simulink model "ModeAdjust"  (R2018b)
settings: Solver=FixedStepDiscrete  StartTime=0.0  StopTime=inf  FixedStep=0.01  RelTol=1e-3
undefined symbols (not defined in the file or in its folder): IfKeSMSbSeatMovBkRclnEnable_Val, IfKeSMSbSeatMovFrwdBkwdEnable_Val, IfKeSMSbSeatMovFtrstEnable_Val, IfKeSMSbSeatMovHdrstFrwdBkwdEnable_Val, IfKeSMSbSeatMovHdUpwdDnwdEnable_Val, IfKeSMSbSeatMovLgrstEnable_Val, IfKeSMSbSeatMovLtwdRtwdEnable_Val, IfVeSMSeStNumConfig, KeSMSbArmscreenMovEnable_Val, KeSMSbSeatMovLgrstExpdEnable_Val, KeSMSuFirstRwStBackPosDelta_Val, KeSMSuFirstRwStBackPosTolr_Val, KeSMSuFirstRwStCushFrntPosDelta_Val, KeSMSuFirstRwStCushFrntPosTolr_Val, KeSMSuFirstRwStCushRePosDelta_Val, KeSMSuFirstRwStCushRePosTolr_Val, KeSMSuFirstRwStFootrestPosDelta_Val, KeSMSuFirstRwStFootrestPosTolr_Val, KeSMSuFirstRwStFwdBkwdPosDelta_Val, KeSMSuFirstRwStFwdBkwdPosTolr_Val, KeSMSuMdMotFinshdTm_Val, KeSMSuMdRetryTm1_Val, KeSMSuModeReqDurgTm_Val, KeSMSuSecRwStArmTochPosDelta_Val, KeSMSuSecRwStArmTochPosTolr_Val, KeSMSuSecRwStBackPosDelta_Val, KeSMSuSecRwStBackPosTolr_Val, KeSMSuSecRwStFtrstUpwdDnwdPosDelta_Val, KeSMSuSecRwStFtrstUpwdDnwdPosTolr_Val, KeSMSuSecRwStFwdBkwdPosDelta_Val, KeSMSuSecRwStFwdBkwdPosTolr_Val, KeSMSuSecRwStHeadrestFwdBkwdPosDelta_Val, KeSMSuSecRwStHeadrestFwdBkwdPosTolr_Val, KeSMSuSecRwStHeadrestUpwdDwnwdPosDelta_Val, KeSMSuSecRwStHeadrestUpwdDwnwdPosTolr_Val, KeSMSuSecRwStLegrestInOutPosDelta_Val, KeSMSuSecRwStLegrestInOutPosTolr_Val, KeSMSuSecRwStLegrestUpwdDwnwdPosDelta_Val, KeSMSuSecRwStLegrestUpwdDwnwdPosTolr_Val, KeSMSuSecRwStLwdRwdPosDelta_Val, KeSMSuSecRwStLwdRwdPosTolr_Val, KeSMSuSecRwStVIPFtrstRefAngle_Val, KeSMSuThirdRwStFwdBkwdPosDelta_Val, KeSMSuThirdRwStFwdBkwdPosTolr_Val, KeSMSuThrdRwCushFoldPosDelta_Val, KeSMSuThrdRwCushFoldPosTolr_Val, KeSMSuThrdRwStBackPosDelta_Val, KeSMSuThrdRwStBackPosTolr_Val, KeSMSw4SLegrstCloseMdSecRwLtStFtrstUpwdDnwdPos_Val, KeSMSw4SLegrstCloseMdSecRwLtStFtrstUpwdDnwdPosMax_Val, KeSMSw4SLegrstCloseMdSecRwLtStFtrstUpwdDnwdPosMin_Val, KeSMSw4SLegrstCloseMdSecRwLtStLgrstOtwdInwdPos_Val, KeSMSw4SLegrstCloseMdSecRwLtStLgrstOtwdInwdPosMax_Val, KeSMSw4SLegrstCloseMdSecRwLtStLgrstOtwdInwdPosMin_Val, KeSMSw4SLegrstCloseMdSecRwLtStLgrstUpwdDnwdPos_Val, KeSMSw4SLegrstCloseMdSecRwLtStLgrstUpwdDnwdPosMax_Val, KeSMSw4SLegrstCloseMdSecRwLtStLgrstUpwdDnwdPosMin_Val, KeSMSw4SLegrstCloseMdSecRwRtStFtrstUpwdDnwdPos_Val, KeSMSw4SLegrstCloseMdSecRwRtStFtrstUpwdDnwdPosMax_Val, KeSMSw4SLegrstCloseMdSecRwRtStFtrstUpwdDnwdPosMin_Val ... (+1138)
libraries: Lib x401
(part 33 of 35)

== system ModeAdjust/ModeAdjustRunnable_sys/ModeAdjust/ArrivedAtTargetPosChk/Vip4s/R2Rt ==
  SecRwLtStsPoss : Inport
  ModeStCalib_2L : Inport  Port=2
  StConfig : Inport  Port=3
  SecRwLtStsPoss4s : Inport  Port=4
  StConfig4s : Inport  Port=5
  SecRwRtStPossV : Inport  Port=6
  PosV4s : Inport  Port=7
  Rt4sHightIndex : Inport  Port=8
  PosDeltaCalib : Inport  Port=9
  Bus Creator{1..7} (7 alike) : BusCreator  Inputs=9
  Bus Selector : BusSelector  OutputSignals=IfVeSMSuSecRwRtStBkReclnUpwdDnwdPos_Val_read,IfVeSMSuSecRwRtStFrwdBkwdPos_Val_read,IfVeSMSuSecRwRtStHPassStUpwdDnwdPos_Val_read,IfVeSMSuSecRwRtStLgrstUpwdDnwdPos_Val_read,IfVeSMSuSecRwRtStLtwdRtwdPos_Val_read,SecRwRtStArmScrnPos_Val_read
  Bus Selector1 : BusSelector  OutputSignals=IfVeSMSuSecRwRtStLgrstOtwdInwdPos_Val_read,IfVeSMSuRrRtStFtUpwdDnwdPos_Val_read,IfVeSMSuSecRwRtStHdrstFrwdBkwdPos_Val_read
  Bus Selector2 : BusSelector  OutputSignals=BkReclnUpwdDnwdPos,BkReclnUpwdDnwdPosMax,BkReclnUpwdDnwdPosMin,LgrstUpwdPos,LgrstUpwdPosMax,LgrstUpwdPosMin,FtrstUpwdDnwdPos,FtrstUpwdDnwdPosMax,FtrstUpwdDnwdPosMin
  Bus Selector3 : BusSelector  OutputSignals=VipRSecRwRtSt
  Bus Selector4 : BusSelector  OutputSignals=BkReclnUpwdDnwdMovConfig,ArmTouchMovConfig,FrwdBkwdMovConfig,LgrstUpwdMovConfig,LtwdRtwdMovConfig
  Bus Selector5 : BusSelector  OutputSignals=LgrstExpdMovConfig,FtrstMovConfig,HdrstUpwdDnwdMovConfig,HdrstFrwdBkwdMovConfig
  Bus Selector6 : BusSelector  OutputSignals=IfVeSMSuSecRwRtStBkReclnUpwdDnwdPosV_Val_read,IfVeSMSuSecRwRtStFrwdBkwdPosV_Val_read,IfVeSMSuSecRwRtStHPassStUpwdDnwdPosV_Val_read,IfVeSMSuSecRwRtStLgrstUpwdDnwdPosV_Val_read,IfVeSMSuSecRwRtStLtwdRtwdPosV_Val_read,SecRwRtStArmScrnPosV_Val_read
  Bus Selector7 : BusSelector  OutputSignals=IfVeSMSuSecRwRtStLgrstOtwdInwdPosV_Val_read,IfVeSMSuRrRtStFtUpwdDnwdPosV_Val_read,IfVeSMSuSecRwRtStHdrstFrwdBkwdPosV_Val_read
  Bus Selector8 : BusSelector  OutputSignals=HdrstUpwdDnwdPosMax,HdrstUpwdDnwdPosMin,LgrstOtwdInwdPosMax,LgrstOtwdInwdPosMin,HdrstFrwdBkwdnwdPosMax,HdrstFrwdBkwdnwdPosMin
  Bus Selector9 : BusSelector  OutputSignals=KeSMSuSecRwStHeadrestFwdBkwdPosDelta_Val,KeSMSuSecRwStHeadrestUpwdDwnwdPosDelta_Val,KeSMSuSecRwStLegrestInOutPosDelta_Val,KeSMSuSecRwStFtrstUpwdDnwdPosDelta_Val,KeSMSuSecRwStBackPosDelta_Val,KeSMSuSecRwStLegrestUpwdDwnwdPosDelta_Val
  CheckAtPos{,1..5} (6 alike) : Lib/CheckAtPos  SystemSampleTime=-1
  Constant{1..12} (12 alike) : Constant  Value=0  OutDataTypeStr=boolean
  IsArrivedTarZone{,1..5} (6 alike) : Lib/CommonUsed/IniPosjudg/Subsystem2  SystemSampleTime=-1
  Logical Operator9 : Logic  Inputs=6  AllPortsSameDT=off  OutDataTypeStr=boolean
  Multiport Switch : MultiPortSwitch  DataPortOrder=Zero-based contiguous  Inputs=7  DiagnosticForDefault=None  zeroidx=on
  PA_KeSMSw4sVIPMDSecRwRtStHdrstFrwdBkwdPosMax_160_Val : Constant  Value=KeSMSw4sVIPMDSecRwRtStHdrstFrwdBkwdPosMax_160_Val
  PA_KeSMSw4sVIPMDSecRwRtStHdrstFrwdBkwdPosMax_165_Val : Constant  Value=KeSMSw4sVIPMDSecRwRtStHdrstFrwdBkwdPosMax_165_Val
  PA_KeSMSw4sVIPMDSecRwRtStHdrstFrwdBkwdPosMax_170_Val : Constant  Value=KeSMSw4sVIPMDSecRwRtStHdrstFrwdBkwdPosMax_170_Val
  PA_KeSMSw4sVIPMDSecRwRtStHdrstFrwdBkwdPosMax_175_Val : Constant  Value=KeSMSw4sVIPMDSecRwRtStHdrstFrwdBkwdPosMax_175_Val
  PA_KeSMSw4sVIPMDSecRwRtStHdrstFrwdBkwdPosMax_180_Val : Constant  Value=KeSMSw4sVIPMDSecRwRtStHdrstFrwdBkwdPosMax_180_Val
  PA_KeSMSw4sVIPMDSecRwRtStHdrstFrwdBkwdPosMax_Below160_Val : Constant  Value=KeSMSw4sVIPMDSecRwRtStHdrstFrwdBkwdPosMax_Below160_Val
  PA_KeSMSw4sVIPMDSecRwRtStHdrstFrwdBkwdPosMax_Over180_Val : Constant  Value=KeSMSw4sVIPMDSecRwRtStHdrstFrwdBkwdPosMax_Over180_Val
  PA_KeSMSw4sVIPMDSecRwRtStHdrstFrwdBkwdPosMin_160_Val : Constant  Value=KeSMSw4sVIPMDSecRwRtStHdrstFrwdBkwdPosMin_160_Val
  PA_KeSMSw4sVIPMDSecRwRtStHdrstFrwdBkwdPosMin_165_Val : Constant  Value=KeSMSw4sVIPMDSecRwRtStHdrstFrwdBkwdPosMin_165_Val
  PA_KeSMSw4sVIPMDSecRwRtStHdrstFrwdBkwdPosMin_170_Val : Constant  Value=KeSMSw4sVIPMDSecRwRtStHdrstFrwdBkwdPosMin_170_Val
  PA_KeSMSw4sVIPMDSecRwRtStHdrstFrwdBkwdPosMin_175_Val : Constant  Value=KeSMSw4sVIPMDSecRwRtStHdrstFrwdBkwdPosMin_175_Val
  PA_KeSMSw4sVIPMDSecRwRtStHdrstFrwdBkwdPosMin_180_Val : Constant  Value=KeSMSw4sVIPMDSecRwRtStHdrstFrwdBkwdPosMin_180_Val
  PA_KeSMSw4sVIPMDSecRwRtStHdrstFrwdBkwdPosMin_Below160_Val : Constant  Value=KeSMSw4sVIPMDSecRwRtStHdrstFrwdBkwdPosMin_Below160_Val
  PA_KeSMSw4sVIPMDSecRwRtStHdrstFrwdBkwdPosMin_Over180_Val : Constant  Value=KeSMSw4sVIPMDSecRwRtStHdrstFrwdBkwdPosMin_Over180_Val
  PA_KeSMSw4sVIPMDSecRwRtStHdrstFrwdBkwdPos_160_Val : Constant  Value=KeSMSw4sVIPMDSecRwRtStHdrstFrwdBkwdPos_160_Val
  PA_KeSMSw4sVIPMDSecRwRtStHdrstFrwdBkwdPos_165_Val : Constant  Value=KeSMSw4sVIPMDSecRwRtStHdrstFrwdBkwdPos_165_Val
  PA_KeSMSw4sVIPMDSecRwRtStHdrstFrwdBkwdPos_170_Val : Constant  Value=KeSMSw4sVIPMDSecRwRtStHdrstFrwdBkwdPos_170_Val
  PA_KeSMSw4sVIPMDSecRwRtStHdrstFrwdBkwdPos_175_Val : Constant  Value=KeSMSw4sVIPMDSecRwRtStHdrstFrwdBkwdPos_175_Val
  PA_KeSMSw4sVIPMDSecRwRtStHdrstFrwdBkwdPos_180_Val : Constant  Value=KeSMSw4sVIPMDSecRwRtStHdrstFrwdBkwdPos_180_Val
  PA_KeSMSw4sVIPMDSecRwRtStHdrstFrwdBkwdPos_Below160_Val : Constant  Value=KeSMSw4sVIPMDSecRwRtStHdrstFrwdBkwdPos_Below160_Val
  PA_KeSMSw4sVIPMDSecRwRtStHdrstFrwdBkwdPos_Over180_Val : Constant  Value=KeSMSw4sVIPMDSecRwRtStHdrstFrwdBkwdPos_Over180_Val
  PA_KeSMSw4sVIPMDSecRwRtStHdrstUpwdPosMax_160_Val : Constant  Value=KeSMSw4sVIPMDSecRwRtStHdrstUpwdPosMax_160_Val
  PA_KeSMSw4sVIPMDSecRwRtStHdrstUpwdPosMax_165_Val : Constant  Value=KeSMSw4sVIPMDSecRwRtStHdrstUpwdPosMax_165_Val
  PA_KeSMSw4sVIPMDSecRwRtStHdrstUpwdPosMax_170_Val : Constant  Value=KeSMSw4sVIPMDSecRwRtStHdrstUpwdPosMax_170_Val
  PA_KeSMSw4sVIPMDSecRwRtStHdrstUpwdPosMax_175_Val : Constant  Value=KeSMSw4sVIPMDSecRwRtStHdrstUpwdPosMax_175_Val
  PA_KeSMSw4sVIPMDSecRwRtStHdrstUpwdPosMax_180_Val : Constant  Value=KeSMSw4sVIPMDSecRwRtStHdrstUpwdPosMax_180_Val
  PA_KeSMSw4sVIPMDSecRwRtStHdrstUpwdPosMax_Below160_Val : Constant  Value=KeSMSw4sVIPMDSecRwRtStHdrstUpwdPosMax_Below160_Val
  PA_KeSMSw4sVIPMDSecRwRtStHdrstUpwdPosMax_Over180_Val : Constant  Value=KeSMSw4sVIPMDSecRwRtStHdrstUpwdPosMax_Over180_Val
  PA_KeSMSw4sVIPMDSecRwRtStHdrstUpwdPosMin_160_Val : Constant  Value=KeSMSw4sVIPMDSecRwRtStHdrstUpwdPosMin_160_Val
  PA_KeSMSw4sVIPMDSecRwRtStHdrstUpwdPosMin_165_Val : Constant  Value=KeSMSw4sVIPMDSecRwRtStHdrstUpwdPosMin_165_Val
  PA_KeSMSw4sVIPMDSecRwRtStHdrstUpwdPosMin_170_Val : Constant  Value=KeSMSw4sVIPMDSecRwRtStHdrstUpwdPosMin_170_Val
  PA_KeSMSw4sVIPMDSecRwRtStHdrstUpwdPosMin_175_Val : Constant  Value=KeSMSw4sVIPMDSecRwRtStHdrstUpwdPosMin_175_Val
  PA_KeSMSw4sVIPMDSecRwRtStHdrstUpwdPosMin_180_Val : Constant  Value=KeSMSw4sVIPMDSecRwRtStHdrstUpwdPosMin_180_Val
  PA_KeSMSw4sVIPMDSecRwRtStHdrstUpwdPosMin_Below160_Val : Constant  Value=KeSMSw4sVIPMDSecRwRtStHdrstUpwdPosMin_Below160_Val
  PA_KeSMSw4sVIPMDSecRwRtStHdrstUpwdPosMin_Over180_Val : Constant  Value=KeSMSw4sVIPMDSecRwRtStHdrstUpwdPosMin_Over180_Val
  PA_KeSMSw4sVIPMDSecRwRtStHdrstUpwdPos_160_Val : Constant  Value=KeSMSw4sVIPMDSecRwRtStHdrstUpwdPos_160_Val
  PA_KeSMSw4sVIPMDSecRwRtStHdrstUpwdPos_165_Val : Constant  Value=KeSMSw4sVIPMDSecRwRtStHdrstUpwdPos_165_Val
  PA_KeSMSw4sVIPMDSecRwRtStHdrstUpwdPos_170_Val : Constant  Value=KeSMSw4sVIPMDSecRwRtStHdrstUpwdPos_170_Val
  PA_KeSMSw4sVIPMDSecRwRtStHdrstUpwdPos_175_Val : Constant  Value=KeSMSw4sVIPMDSecRwRtStHdrstUpwdPos_175_Val
  PA_KeSMSw4sVIPMDSecRwRtStHdrstUpwdPos_180_Val : Constant  Value=KeSMSw4sVIPMDSecRwRtStHdrstUpwdPos_180_Val
  PA_KeSMSw4sVIPMDSecRwRtStHdrstUpwdPos_Below160_Val : Constant  Value=KeSMSw4sVIPMDSecRwRtStHdrstUpwdPos_Below160_Val
  PA_KeSMSw4sVIPMDSecRwRtStHdrstUpwdPos_Over180_Val : Constant  Value=KeSMSw4sVIPMDSecRwRtStHdrstUpwdPos_Over180_Val
  PA_KeSMSw4sVIPMDSecRwRtStLgrstOtwdInwdPosMax_160_Val : Constant  Value=KeSMSw4sVIPMDSecRwRtStLgrstOtwdInwdPosMax_160_Val
  PA_KeSMSw4sVIPMDSecRwRtStLgrstOtwdInwdPosMax_165_Val : Constant  Value=KeSMSw4sVIPMDSecRwRtStLgrstOtwdInwdPosMax_165_Val
  PA_KeSMSw4sVIPMDSecRwRtStLgrstOtwdInwdPosMax_170_Val : Constant  Value=KeSMSw4sVIPMDSecRwRtStLgrstOtwdInwdPosMax_170_Val
  PA_KeSMSw4sVIPMDSecRwRtStLgrstOtwdInwdPosMax_175_Val : Constant  Value=KeSMSw4sVIPMDSecRwRtStLgrstOtwdInwdPosMax_175_Val
  PA_KeSMSw4sVIPMDSecRwRtStLgrstOtwdInwdPosMax_180_Val : Constant  Value=KeSMSw4sVIPMDSecRwRtStLgrstOtwdInwdPosMax_180_Val
  PA_KeSMSw4sVIPMDSecRwRtStLgrstOtwdInwdPosMax_Below160_Val : Constant  Value=KeSMSw4sVIPMDSecRwRtStLgrstOtwdInwdPosMax_Below160_Val
  PA_KeSMSw4sVIPMDSecRwRtStLgrstOtwdInwdPosMax_Over180_Val : Constant  Value=KeSMSw4sVIPMDSecRwRtStLgrstOtwdInwdPosMax_Over180_Val
  PA_KeSMSw4sVIPMDSecRwRtStLgrstOtwdInwdPosMin_160_Val : Constant  Value=KeSMSw4sVIPMDSecRwRtStLgrstOtwdInwdPosMin_160_Val
  PA_KeSMSw4sVIPMDSecRwRtStLgrstOtwdInwdPosMin_165_Val : Constant  Value=KeSMSw4sVIPMDSecRwRtStLgrstOtwdInwdPosMin_165_Val
  PA_KeSMSw4sVIPMDSecRwRtStLgrstOtwdInwdPosMin_170_Val : Constant  Value=KeSMSw4sVIPMDSecRwRtStLgrstOtwdInwdPosMin_170_Val
  PA_KeSMSw4sVIPMDSecRwRtStLgrstOtwdInwdPosMin_175_Val : Constant  Value=KeSMSw4sVIPMDSecRwRtStLgrstOtwdInwdPosMin_175_Val
  PA_KeSMSw4sVIPMDSecRwRtStLgrstOtwdInwdPosMin_180_Val : Constant  Value=KeSMSw4sVIPMDSecRwRtStLgrstOtwdInwdPosMin_180_Val
  PA_KeSMSw4sVIPMDSecRwRtStLgrstOtwdInwdPosMin_Below160_Val : Constant  Value=KeSMSw4sVIPMDSecRwRtStLgrstOtwdInwdPosMin_Below160_Val
  PA_KeSMSw4sVIPMDSecRwRtStLgrstOtwdInwdPosMin_Over180_Val : Constant  Value=KeSMSw4sVIPMDSecRwRtStLgrstOtwdInwdPosMin_Over180_Val
  PA_KeSMSw4sVIPMDSecRwRtStLgrstOtwdInwdPos_160_Val : Constant  Value=KeSMSw4sVIPMDSecRwRtStLgrstOtwdInwdPos_160_Val
  PA_KeSMSw4sVIPMDSecRwRtStLgrstOtwdInwdPos_165_Val : Constant  Value=KeSMSw4sVIPMDSecRwRtStLgrstOtwdInwdPos_165_Val
  PA_KeSMSw4sVIPMDSecRwRtStLgrstOtwdInwdPos_170_Val : Constant  Value=KeSMSw4sVIPMDSecRwRtStLgrstOtwdInwdPos_170_Val
  PA_KeSMSw4sVIPMDSecRwRtStLgrstOtwdInwdPos_175_Val : Constant  Value=KeSMSw4sVIPMDSecRwRtStLgrstOtwdInwdPos_175_Val
  PA_KeSMSw4sVIPMDSecRwRtStLgrstOtwdInwdPos_180_Val : Constant  Value=KeSMSw4sVIPMDSecRwRtStLgrstOtwdInwdPos_180_Val
  PA_KeSMSw4sVIPMDSecRwRtStLgrstOtwdInwdPos_Below160_Val : Constant  Value=KeSMSw4sVIPMDSecRwRtStLgrstOtwdInwdPos_Below160_Val
  PA_KeSMSw4sVIPMDSecRwRtStLgrstOtwdInwdPos_Over180_Val : Constant  Value=KeSMSw4sVIPMDSecRwRtStLgrstOtwdInwdPos_Over180_Val
  R2Lt_ArrivedTarPos : Outport
  Calib_VIP4sRAdpt : Outport  Port=2
  wires:
  IsArrivedTarZone/1 -> [Step1_1_ArrivedTarPos]
  [SecRwLtStBkReclnUpwdDnwdPos] -> IsArrivedTarZone/1
  [K_BkReclnUpwdDnwdPosMin] -> IsArrivedTarZone/2
  Bus Selector/5 -> [SecRwLtStLtwdRtwdPos]  "<IfVeSMSuSecRwRtStLtwdRtwdPos_Val_read>"
  SecRwLtStsPoss/1 -> Bus Selector/1
  Bus Selector/3 -> [SecRwLtStHPassStUpwdDnwdPos]  "<IfVeSMSuSecRwRtStHPassStUpwdDnwdPos_Val_read>"
  Bus Selector/4 -> [SecRwLtStLgrstUpwdDnwdPos]  "<IfVeSMSuSecRwRtStLgrstUpwdDnwdPos_Val_read>"
  Bus Selector/2 -> [SecRwLtStFrwdBkwdPos]  "<IfVeSMSuSecRwRtStFrwdBkwdPos_Val_read>"
  Bus Selector/1 -> [SecRwLtStBkReclnUpwdDnwdPos]  "<IfVeSMSuSecRwRtStBkReclnUpwdDnwdPos_Val_read>"
  [K_LgrstUpwdPosMin] -> IsArrivedTarZone1/2
  [SecRwLtStLgrstUpwdDnwdPos] -> IsArrivedTarZone1/1
  IsArrivedTarZone1/1 -> [Step1_2_ArrivedTarPos]
  Logical Operator9/1 -> R2Lt_ArrivedTarPos/1
  IsArrivedTarZone2/1 -> [Step1_3_ArrivedTarPos]
  Bus Selector/6 -> [SecRwLtStArmScrnPos]  "<SecRwRtStArmScrnPos_Val_read>"
  [KeSMSuSecRwStBackPosDelta_Val] -> IsArrivedTarZone/3
  [K_BkReclnUpwdDnwdPosMax] -> IsArrivedTarZone/4
  [K_LgrstUpwdPosMax] -> IsArrivedTarZone1/4
  [KeSMSuSecRwStLegrestUpwdDwnwdPosDelta_Val] -> IsArrivedTarZone1/3
  Bus Selector2/6 -> [K_LgrstUpwdPosMin]  "<LgrstUpwdPosMin>"
  Bus Selector2/4 -> [K_LgrstUpwdPos]  "<LgrstUpwdPos>"
  Bus Selector2/5 -> [K_LgrstUpwdPosMax]  "<LgrstUpwdPosMax>"
  Bus Selector2/1 -> [K_BkReclnUpwdDnwdPos]  "<BkReclnUpwdDnwdPos>"
  Bus Selector2/2 -> [K_BkReclnUpwdDnwdPosMax]  "<BkReclnUpwdDnwdPosMax>"
  Bus Selector3/1 -> Bus Selector2/1  "<VipRSecRwRtSt>"
  Bus Selector2/3 -> [K_BkReclnUpwdDnwdPosMin]  "<BkReclnUpwdDnwdPosMin>"
  ModeStCalib_2L/1 -> Bus Selector3/1
  StConfig/1 -> Bus Selector4/1
  Bus Selector4/3 -> [FrwdBkwdMovConfig]  "<FrwdBkwdMovConfig>"
  Bus Selector4/5 -> [LtwdRtwdMovConfig]  "<LtwdRtwdMovConfig>"
  Bus Selector4/4 -> [LgrstUpwdMovConfig]  "<LgrstUpwdMovConfig>"
  Bus Selector4/2 -> [ArmTouchMovConfig]  "<ArmTouchMovConfig>"
  Bus Selector4/1 -> [BkReclnUpwdDnwdMovConfig]  "<BkReclnUpwdDnwdMovConfig>"
  [K_HdrstUpwdPosMax] -> IsArrivedTarZone2/4
  [K_HdrstUpwdPosMin] -> IsArrivedTarZone2/2
  [SecRwLtStHPassStUpwdDnwdPos] -> IsArrivedTarZone2/1
  [KeSMSuSecRwStHeadrestUpwdDwnwdPosDelta_Val] -> IsArrivedTarZone2/3
  [KeSMSuSecRwStFtrstUpwdDnwdPosDelta_Val] -> IsArrivedTarZone3/3
  SecRwLtStsPoss4s/1 -> Bus Selector1/1
  Bus Selector1/1 -> [SecRwLtStLgrstOtwdInwdPos]  "<IfVeSMSuSecRwRtStLgrstOtwdInwdPos_Val_read>"
  Bus Selector1/2 -> [IfVeSMSuRrLtStFtUpwdDnwdPos]  "<IfVeSMSuRrRtStFtUpwdDnwdPos_Val_read>"
  [IfVeSMSuRrLtStFtUpwdDnwdPos] -> IsArrivedTarZone3/1
  Bus Selector2/7 -> [K_FtrstUpwdDnwdPos]  "<FtrstUpwdDnwdPos>"
  Bus Selector2/8 -> [K_FtrstUpwdDnwdPos_Max]  "<FtrstUpwdDnwdPosMax>"
  Bus Selector2/9 -> [K_FtrstUpwdDnwdPos_Min]  "<FtrstUpwdDnwdPosMin>"
  [K_FtrstUpwdDnwdPos_Min] -> IsArrivedTarZone3/2
  [K_FtrstUpwdDnwdPos_Max] -> IsArrivedTarZone3/4
  IsArrivedTarZone3/1 -> [Step1_4_ArrivedTarPos]
  [K_LgrstOtwdInwdPos_Min] -> IsArrivedTarZone4/2
  [K_LgrstOtwdInwdPos_Max] -> IsArrivedTarZone4/4
  [SecRwLtStLgrstOtwdInwdPos] -> IsArrivedTarZone4/1
  [KeSMSuSecRwStLegrestInOutPosDelta_Val] -> IsArrivedTarZone4/3
  IsArrivedTarZone4/1 -> [Step1_5_ArrivedTarPos]
  StConfig4s/1 -> Bus Selector5/1
  Bus Selector5/3 -> [HdrstMovConfig]  "<HdrstUpwdDnwdMovConfig>"
  Bus Selector5/1 -> [LgrstExpdMovConfig]  "<LgrstExpdMovConfig>"
  Bus Selector5/2 -> [FtrstMovConfig]  "<FtrstMovConfig>"
  PosV4s/1 -> Bus Selector7/1
  Bus Selector7/2 -> [RrLtStFtUpwdDnwdPosV]  "<IfVeSMSuRrRtStFtUpwdDnwdPosV_Val_read>"
  Bus Selector7/1 -> [SecRwLtStLgrstOtwdInwdPosV]  "<IfVeSMSuSecRwRtStLgrstOtwdInwdPosV_Val_read>"
  Bus Selector6/5 -> [SecRwRtStLtwdRtwdPosV]  "<IfVeSMSuSecRwRtStLtwdRtwdPosV_Val_read>"
  SecRwRtStPossV/1 -> Bus Selector6/1
  Bus Selector6/6 -> [SecRwRtStArmScrnPosV]  "<SecRwRtStArmScrnPosV_Val_read>"
  Bus Selector6/3 -> [SecRwRtStHPassStUpwdDnwdPosV]  "<IfVeSMSuSecRwRtStHPassStUpwdDnwdPosV_Val_read>"
  Bus Selector6/4 -> [SecRwRtStLgrstUpwdDnwdPosV]  "<IfVeSMSuSecRwRtStLgrstUpwdDnwdPosV_Val_read>"
  Bus Selector6/2 -> [SecRwRtStFrwdBkwdPosV]  "<IfVeSMSuSecRwRtStFrwdBkwdPosV_Val_read>"
  Bus Selector6/1 -> [SecRwRtStBkReclnUpwdDnwdPosV]  "<IfVeSMSuSecRwRtStBkReclnUpwdDnwdPosV_Val_read>"
  CheckAtPos2/1 -> Logical Operator9/3  "Vip4sR_Step1_3_ArrivedTarPos"
  CheckAtPos1/1 -> Logical Operator9/2  "Vip4sR_Step1_2_ArrivedTarPos"
  CheckAtPos3/1 -> Logical Operator9/4  "Vip4sR_Step1_4_ArrivedTarPos"
  CheckAtPos/1 -> Logical Operator9/1  "Vip4sR_Step1_1_ArrivedTarPos"
  CheckAtPos4/1 -> Logical Operator9/5  "Vip4sR_Step1_5_ArrivedTarPos"
  [BkReclnUpwdDnwdMovConfig] -> CheckAtPos/1
  [Step1_1_ArrivedTarPos] -> CheckAtPos/3
  [LgrstUpwdMovConfig] -> CheckAtPos1/1
  [Step1_2_ArrivedTarPos] -> CheckAtPos1/3
  [HdrstMovConfig] -> CheckAtPos2/1
  [Step1_3_ArrivedTarPos] -> CheckAtPos2/3
  [FtrstMovConfig] -> CheckAtPos3/1
  [Step1_4_ArrivedTarPos] -> CheckAtPos3/3
  [LgrstExpdMovConfig] -> CheckAtPos4/1
  [Step1_5_ArrivedTarPos] -> CheckAtPos4/3
  Constant8/1 -> CheckAtPos4/4
  Constant7/1 -> CheckAtPos4/5
  Constant2/1 -> CheckAtPos3/4
  Constant1/1 -> CheckAtPos3/5
  Constant4/1 -> CheckAtPos2/4
  Constant3/1 -> CheckAtPos2/5
  Constant6/1 -> CheckAtPos1/4
  Constant5/1 -> CheckAtPos1/5
  Constant12/1 -> CheckAtPos/4
  Constant11/1 -> CheckAtPos/5
  [SecRwRtStBkReclnUpwdDnwdPosV] -> CheckAtPos/2
  [SecRwRtStLgrstUpwdDnwdPosV] -> CheckAtPos1/2
  [SecRwRtStHPassStUpwdDnwdPosV] -> CheckAtPos2/2
  [RrLtStFtUpwdDnwdPosV] -> CheckAtPos3/2
  [SecRwLtStLgrstOtwdInwdPosV] -> CheckAtPos4/2
  Bus Selector5/4 -> [HdrstFrwdBkwdMovConfig]  "<HdrstFrwdBkwdMovConfig>"
  [SecRwRtStHdrstFrwdBkwdPos] -> IsArrivedTarZone5/1
  [HdrstFrwdBkwdMovConfig] -> CheckAtPos5/1
  [Step1_6_ArrivedTarPos] -> CheckAtPos5/3
  IsArrivedTarZone5/1 -> [Step1_6_ArrivedTarPos]
  CheckAtPos5/1 -> Logical Operator9/6  "Vip4sR_Step1_6_ArrivedTarPos"
  [KeSMSuSecRwStHeadrestFwdBkwdPosDelta_Val] -> IsArrivedTarZone5/3
  Constant9/1 -> CheckAtPos5/5
  [K_HdrstFrwdBkwdnwdPosMin] -> IsArrivedTarZone5/2
  [K_HdrstFrwdBkwdnwdPosMax] -> IsArrivedTarZone5/4
  [SecRwRtStHdrstFrwdBkwdPosV] -> CheckAtPos5/2
  Constant10/1 -> CheckAtPos5/4
  Bus Selector7/3 -> [SecRwRtStHdrstFrwdBkwdPosV]  "<IfVeSMSuSecRwRtStHdrstFrwdBkwdPosV_Val_read>"
  Bus Selector1/3 -> [SecRwRtStHdrstFrwdBkwdPos]  "<IfVeSMSuSecRwRtStHdrstFrwdBkwdPos_Val_read>"
  Rt4sHightIndex/1 -> Multiport Switch/1
  Bus Selector8/3 -> [K_LgrstOtwdInwdPos_Max]  "<LgrstOtwdInwdPosMax>"
  Bus Selector8/2 -> [K_HdrstUpwdPosMin]  "<HdrstUpwdDnwdPosMin>"
  Bus Selector8/4 -> [K_LgrstOtwdInwdPos_Min]  "<LgrstOtwdInwdPosMin>"
  Multiport Switch/1 -> Bus Selector8/1, Calib_VIP4sRAdpt/1
  Bus Selector8/1 -> [K_HdrstUpwdPosMax]  "<HdrstUpwdDnwdPosMax>"
  Bus Creator7/1 -> Multiport Switch/2  "VIP4sRAdpt"
  PA_KeSMSw4sVIPMDSecRwRtStLgrstOtwdInwdPosMax_Below160_Val/1 -> Bus Creator7/5  "LgrstOtwdInwdPosMax"
  PA_KeSMSw4sVIPMDSecRwRtStHdrstUpwdPosMax_Below160_Val/1 -> Bus Creator7/2  "HdrstUpwdDnwdPosMax"
  PA_KeSMSw4sVIPMDSecRwRtStHdrstUpwdPosMin_Below160_Val/1 -> Bus Creator7/3  "HdrstUpwdDnwdPosMin"
  PA_KeSMSw4sVIPMDSecRwRtStHdrstFrwdBkwdPos_Below160_Val/1 -> Bus Creator7/7  "HdrstFrwdBkwdnwdPos"
  PA_KeSMSw4sVIPMDSecRwRtStLgrstOtwdInwdPosMin_Below160_Val/1 -> Bus Creator7/6  "LgrstOtwdInwdPosMin"
  PA_KeSMSw4sVIPMDSecRwRtStHdrstUpwdPos_Below160_Val/1 -> Bus Creator7/1  "HdrstUpwdDnwdPos"
  PA_KeSMSw4sVIPMDSecRwRtStHdrstFrwdBkwdPosMax_Below160_Val/1 -> Bus Creator7/8  "HdrstFrwdBkwdnwdPosMax"
  PA_KeSMSw4sVIPMDSecRwRtStHdrstFrwdBkwdPosMin_Below160_Val/1 -> Bus Creator7/9  "HdrstFrwdBkwdnwdPosMin"
  PA_KeSMSw4sVIPMDSecRwRtStLgrstOtwdInwdPos_Below160_Val/1 -> Bus Creator7/4  "LgrstOtwdInwdPos"
  PA_KeSMSw4sVIPMDSecRwRtStHdrstFrwdBkwdPosMax_160_Val/1 -> Bus Creator1/8  "HdrstFrwdBkwdnwdPosMax"
  PA_KeSMSw4sVIPMDSecRwRtStHdrstFrwdBkwdPos_160_Val/1 -> Bus Creator1/7  "HdrstFrwdBkwdnwdPos"
  PA_KeSMSw4sVIPMDSecRwRtStHdrstFrwdBkwdPosMin_160_Val/1 -> Bus Creator1/9  "HdrstFrwdBkwdnwdPosMin"
  Bus Creator1/1 -> Multiport Switch/3  "VIP4sRAdpt"
  PA_KeSMSw4sVIPMDSecRwRtStHdrstUpwdPosMin_160_Val/1 -> Bus Creator1/3  "HdrstUpwdDnwdPosMin"
  PA_KeSMSw4sVIPMDSecRwRtStLgrstOtwdInwdPosMax_160_Val/1 -> Bus Creator1/5  "LgrstOtwdInwdPosMax"
  PA_KeSMSw4sVIPMDSecRwRtStHdrstUpwdPosMax_160_Val/1 -> Bus Creator1/2  "HdrstUpwdDnwdPosMax"
  PA_KeSMSw4sVIPMDSecRwRtStHdrstUpwdPos_160_Val/1 -> Bus Creator1/1  "HdrstUpwdDnwdPos"
  PA_KeSMSw4sVIPMDSecRwRtStLgrstOtwdInwdPosMin_160_Val/1 -> Bus Creator1/6  "LgrstOtwdInwdPosMin"
  PA_KeSMSw4sVIPMDSecRwRtStLgrstOtwdInwdPos_160_Val/1 -> Bus Creator1/4  "LgrstOtwdInwdPos"
  PA_KeSMSw4sVIPMDSecRwRtStHdrstFrwdBkwdPosMax_165_Val/1 -> Bus Creator2/8  "HdrstFrwdBkwdnwdPosMax"
  PA_KeSMSw4sVIPMDSecRwRtStHdrstFrwdBkwdPos_165_Val/1 -> Bus Creator2/7  "HdrstFrwdBkwdnwdPos"
  PA_KeSMSw4sVIPMDSecRwRtStHdrstFrwdBkwdPosMin_165_Val/1 -> Bus Creator2/9  "HdrstFrwdBkwdnwdPosMin"
  Bus Creator2/1 -> Multiport Switch/4  "VIP4sRAdpt"
  PA_KeSMSw4sVIPMDSecRwRtStHdrstUpwdPosMin_165_Val/1 -> Bus Creator2/3  "HdrstUpwdDnwdPosMin"
  PA_KeSMSw4sVIPMDSecRwRtStLgrstOtwdInwdPosMax_165_Val/1 -> Bus Creator2/5  "LgrstOtwdInwdPosMax"
  PA_KeSMSw4sVIPMDSecRwRtStHdrstUpwdPosMax_165_Val/1 -> Bus Creator2/2  "HdrstUpwdDnwdPosMax"
  PA_KeSMSw4sVIPMDSecRwRtStHdrstUpwdPos_165_Val/1 -> Bus Creator2/1  "HdrstUpwdDnwdPos"
  PA_KeSMSw4sVIPMDSecRwRtStLgrstOtwdInwdPosMin_165_Val/1 -> Bus Creator2/6  "LgrstOtwdInwdPosMin"
  PA_KeSMSw4sVIPMDSecRwRtStLgrstOtwdInwdPos_165_Val/1 -> Bus Creator2/4  "LgrstOtwdInwdPos"
  PA_KeSMSw4sVIPMDSecRwRtStHdrstFrwdBkwdPosMax_170_Val/1 -> Bus Creator3/8  "HdrstFrwdBkwdnwdPosMax"
  PA_KeSMSw4sVIPMDSecRwRtStHdrstFrwdBkwdPos_170_Val/1 -> Bus Creator3/7  "HdrstFrwdBkwdnwdPos"
  PA_KeSMSw4sVIPMDSecRwRtStHdrstFrwdBkwdPosMin_170_Val/1 -> Bus Creator3/9  "HdrstFrwdBkwdnwdPosMin"
  Bus Creator3/1 -> Multiport Switch/5  "VIP4sRAdpt"
  PA_KeSMSw4sVIPMDSecRwRtStHdrstUpwdPosMin_170_Val/1 -> Bus Creator3/3  "HdrstUpwdDnwdPosMin"
  PA_KeSMSw4sVIPMDSecRwRtStLgrstOtwdInwdPosMax_170_Val/1 -> Bus Creator3/5  "LgrstOtwdInwdPosMax"
  PA_KeSMSw4sVIPMDSecRwRtStHdrstUpwdPosMax_170_Val/1 -> Bus Creator3/2  "HdrstUpwdDnwdPosMax"
  PA_KeSMSw4sVIPMDSecRwRtStHdrstUpwdPos_170_Val/1 -> Bus Creator3/1  "HdrstUpwdDnwdPos"
  PA_KeSMSw4sVIPMDSecRwRtStLgrstOtwdInwdPosMin_170_Val/1 -> Bus Creator3/6  "LgrstOtwdInwdPosMin"
  PA_KeSMSw4sVIPMDSecRwRtStLgrstOtwdInwdPos_170_Val/1 -> Bus Creator3/4  "LgrstOtwdInwdPos"
  PA_KeSMSw4sVIPMDSecRwRtStHdrstFrwdBkwdPosMax_175_Val/1 -> Bus Creator4/8  "HdrstFrwdBkwdnwdPosMax"
  PA_KeSMSw4sVIPMDSecRwRtStHdrstFrwdBkwdPos_175_Val/1 -> Bus Creator4/7  "HdrstFrwdBkwdnwdPos"
  PA_KeSMSw4sVIPMDSecRwRtStHdrstFrwdBkwdPosMin_175_Val/1 -> Bus Creator4/9  "HdrstFrwdBkwdnwdPosMin"
  Bus Creator4/1 -> Multiport Switch/6  "VIP4sRAdpt"
  PA_KeSMSw4sVIPMDSecRwRtStHdrstUpwdPosMin_175_Val/1 -> Bus Creator4/3  "HdrstUpwdDnwdPosMin"
  PA_KeSMSw4sVIPMDSecRwRtStLgrstOtwdInwdPosMax_175_Val/1 -> Bus Creator4/5  "LgrstOtwdInwdPosMax"
  PA_KeSMSw4sVIPMDSecRwRtStHdrstUpwdPosMax_175_Val/1 -> Bus Creator4/2  "HdrstUpwdDnwdPosMax"
  PA_KeSMSw4sVIPMDSecRwRtStHdrstUpwdPos_175_Val/1 -> Bus Creator4/1  "HdrstUpwdDnwdPos"
  PA_KeSMSw4sVIPMDSecRwRtStLgrstOtwdInwdPosMin_175_Val/1 -> Bus Creator4/6  "LgrstOtwdInwdPosMin"
  PA_KeSMSw4sVIPMDSecRwRtStLgrstOtwdInwdPos_175_Val/1 -> Bus Creator4/4  "LgrstOtwdInwdPos"
  PA_KeSMSw4sVIPMDSecRwRtStHdrstFrwdBkwdPosMax_180_Val/1 -> Bus Creator5/8  "HdrstFrwdBkwdnwdPosMax"
  PA_KeSMSw4sVIPMDSecRwRtStHdrstFrwdBkwdPos_180_Val/1 -> Bus Creator5/7  "HdrstFrwdBkwdnwdPos"
  PA_KeSMSw4sVIPMDSecRwRtStHdrstFrwdBkwdPosMin_180_Val/1 -> Bus Creator5/9  "HdrstFrwdBkwdnwdPosMin"
  Bus Creator5/1 -> Multiport Switch/7  "VIP4sRAdpt"
  PA_KeSMSw4sVIPMDSecRwRtStHdrstUpwdPosMin_180_Val/1 -> Bus Creator5/3  "HdrstUpwdDnwdPosMin"
  PA_KeSMSw4sVIPMDSecRwRtStLgrstOtwdInwdPosMax_180_Val/1 -> Bus Creator5/5  "LgrstOtwdInwdPosMax"
  PA_KeSMSw4sVIPMDSecRwRtStHdrstUpwdPosMax_180_Val/1 -> Bus Creator5/2  "HdrstUpwdDnwdPosMax"
  PA_KeSMSw4sVIPMDSecRwRtStHdrstUpwdPos_180_Val/1 -> Bus Creator5/1  "HdrstUpwdDnwdPos"
  PA_KeSMSw4sVIPMDSecRwRtStLgrstOtwdInwdPosMin_180_Val/1 -> Bus Creator5/6  "LgrstOtwdInwdPosMin"
  PA_KeSMSw4sVIPMDSecRwRtStLgrstOtwdInwdPos_180_Val/1 -> Bus Creator5/4  "LgrstOtwdInwdPos"
  PA_KeSMSw4sVIPMDSecRwRtStHdrstFrwdBkwdPosMax_Over180_Val/1 -> Bus Creator6/8  "HdrstFrwdBkwdnwdPosMax"
  PA_KeSMSw4sVIPMDSecRwRtStHdrstFrwdBkwdPos_Over180_Val/1 -> Bus Creator6/7  "HdrstFrwdBkwdnwdPos"
  PA_KeSMSw4sVIPMDSecRwRtStHdrstFrwdBkwdPosMin_Over180_Val/1 -> Bus Creator6/9  "HdrstFrwdBkwdnwdPosMin"
  Bus Creator6/1 -> Multiport Switch/8  "VIP4sRAdpt"
  PA_KeSMSw4sVIPMDSecRwRtStHdrstUpwdPosMin_Over180_Val/1 -> Bus Creator6/3  "HdrstUpwdDnwdPosMin"
  PA_KeSMSw4sVIPMDSecRwRtStLgrstOtwdInwdPosMax_Over180_Val/1 -> Bus Creator6/5  "LgrstOtwdInwdPosMax"
  PA_KeSMSw4sVIPMDSecRwRtStHdrstUpwdPosMax_Over180_Val/1 -> Bus Creator6/2  "HdrstUpwdDnwdPosMax"
  PA_KeSMSw4sVIPMDSecRwRtStHdrstUpwdPos_Over180_Val/1 -> Bus Creator6/1  "HdrstUpwdDnwdPos"
  PA_KeSMSw4sVIPMDSecRwRtStLgrstOtwdInwdPosMin_Over180_Val/1 -> Bus Creator6/6  "LgrstOtwdInwdPosMin"
  PA_KeSMSw4sVIPMDSecRwRtStLgrstOtwdInwdPos_Over180_Val/1 -> Bus Creator6/4  "LgrstOtwdInwdPos"
  Bus Selector8/5 -> [K_HdrstFrwdBkwdnwdPosMax]  "<HdrstFrwdBkwdnwdPosMax>"
  Bus Selector8/6 -> [K_HdrstFrwdBkwdnwdPosMin]  "<HdrstFrwdBkwdnwdPosMin>"
  Bus Selector9/5 -> [KeSMSuSecRwStBackPosDelta_Val]  "<KeSMSuSecRwStBackPosDelta_Val>"
  Bus Selector9/4 -> [KeSMSuSecRwStFtrstUpwdDnwdPosDelta_Val]  "<KeSMSuSecRwStFtrstUpwdDnwdPosDelta_Val>"
  Bus Selector9/6 -> [KeSMSuSecRwStLegrestUpwdDwnwdPosDelta_Val]  "<KeSMSuSecRwStLegrestUpwdDwnwdPosDelta_Val>"
  Bus Selector9/2 -> [KeSMSuSecRwStHeadrestUpwdDwnwdPosDelta_Val]  "<KeSMSuSecRwStHeadrestUpwdDwnwdPosDelta_Val>"
  Bus Selector9/3 -> [KeSMSuSecRwStLegrestInOutPosDelta_Val]  "<KeSMSuSecRwStLegrestInOutPosDelta_Val>"
  Bus Selector9/1 -> [KeSMSuSecRwStHeadrestFwdBkwdPosDelta_Val]  "<KeSMSuSecRwStHeadrestFwdBkwdPosDelta_Val>"
  PosDeltaCalib/1 -> Bus Selector9/1

== system ModeAdjust/ModeAdjustRunnable_sys/ModeAdjust/VIPL/R2Lt/R2LtSt_BkReclnUpwdDnwd_Lt_Step1 ==
  note: // CurPosV 为0时表示有效，为1时表示无效，数据库中是这么定义的
  MSM_Trig : Inport
  Ena1 : Inport  Port=2
  Ena3 : Inport  Port=3
  Current_Pos : Inport  Port=4
  Calib_Min : Inport  Port=5
  Calib_Max : Inport  Port=6
  Tar_Pos : Inport  Port=7
  Tar_PosDelta : Inport  Port=8
  PosValid : Inport  Port=9
  ChildLocker : Inport  Port=10
  InvalidValue : Inport  Port=11
  Tick : Inport  Port=12
  CheckFinishTm : Inport  Port=13
  StConfig : Inport  Port=14
  InPosJdgModify : Lib/InPosJdgModify  SystemSampleTime=-1
  NOT1 : Logic  Operator=NOT  AllPortsSameDT=off  OutDataTypeStr=boolean
  OR : Logic  Operator=OR  AllPortsSameDT=off  OutDataTypeStr=boolean
  PA_KeSMSuMdRetryTm1_Val : Constant  Value=KeSMSuMdRetryTm1_Val
  PA_KeSMSwDltTrgtPos_Val1 : Constant  Value=0  OutDataTypeStr=boolean
  PA_KeSMSwDltTrgtPos_Val2 : Constant  Value=0  OutDataTypeStr=boolean
  Stg_judg : Lib/CommonUsed/Stg_judg  SystemSampleTime=-1
  Stg_judg1 : Lib/CommonUsed/Stg_judg  SystemSampleTime=-1
  Switch1 : Switch  Criteria=u2 > Threshold
  Switch4 : Switch  Criteria=u2 > Threshold
  isArrivedTarPos1 : Lib/CommonUsed/Subsystem  SystemSampleTime=-1
  ini_st : Outport
  ini_ReclnOverUp : Outport  Port=2
  ini_ReclnOverDwn : Outport  Port=3
  isArrivedTarPos : Outport  Port=4
  TarPos : Outport  Port=5
  Stg_done1 : Outport  Port=6
  Stg_done3 : Outport  Port=7
  wires:
  InvalidValue/1 -> [InvalidValue]
  Ena1/1 -> [Ena1]
  ChildLocker/1 -> [ChildLocker]
  PosValid/1 -> [Valid], Stg_judg/8
  Current_Pos/1 -> Stg_judg/9, Stg_judg1/9, isArrivedTarPos1/1, InPosJdgModify/2
  MSM_Trig/1 -> InPosJdgModify/1
  Calib_Min/1 -> InPosJdgModify/3
  Calib_Max/1 -> InPosJdgModify/4
  InPosJdgModify/1 -> [FrstJudgDone], ini_st/1
  Tar_Pos/1 -> isArrivedTarPos1/2, [tarPos], Stg_judg/4
  Tar_PosDelta/1 -> isArrivedTarPos1/3, InPosJdgModify/5
  isArrivedTarPos1/1 -> isArrivedTarPos/1, [isArrivedTarPos]
  Tick/1 -> Stg_judg1/1, Stg_judg/1
  Stg_judg/2 -> [Stgdone1], Stg_done1/1
  [Ena1] -> Stg_judg/2
  [InvalidValue] -> Stg_judg/3
  OR/1 -> Stg_judg/5
  [ChildLocker] -> Stg_judg/6
  [isArrivedTarPos] -> Stg_judg/7
  Ena3/1 -> [Ena3]
  [Ena3] -> Stg_judg1/2
  [InvalidValue] -> Stg_judg1/3
  [tarPos] -> Stg_judg1/4
  [FrstJudgDone] -> Stg_judg1/5
  [ChildLocker] -> Stg_judg1/6
  [isArrivedTarPos] -> Stg_judg1/7
  [Valid] -> Stg_judg1/8
  Stg_judg1/2 -> [Stgdone3], Stg_done3/1
  Stg_judg/1 -> [TarPos1]
  Stg_judg1/1 -> [TarPos3]
  Switch4/1 -> TarPos/1
  [Ena1] -> Switch4/2
  [TarPos1] -> Switch4/1
  Switch1/1 -> Switch4/3
  [Ena3] -> Switch1/2
  [TarPos3] -> Switch1/1
  [InvalidValue] -> Switch1/3
  InPosJdgModify/3 -> [ini_ReclnOverUp], ini_ReclnOverUp/1
  InPosJdgModify/2 -> ini_ReclnOverDwn/1
  CheckFinishTm/1 -> isArrivedTarPos1/4
  PA_KeSMSwDltTrgtPos_Val1/1 -> Stg_judg1/10
  StConfig/1 -> [StConfig], Stg_judg/11
  [StConfig] -> Stg_judg1/11
  [FrstJudgDone] -> OR/2
  [ini_ReclnOverUp] -> NOT1/1
  NOT1/1 -> OR/1
  PA_KeSMSwDltTrgtPos_Val2/1 -> Stg_judg/10
  [CntLow] -> Stg_judg/12
  [CntLow] -> Stg_judg1/12
  PA_KeSMSuMdRetryTm1_Val/1 -> [CntLow]

== system ModeAdjust/ModeAdjustRunnable_sys/ModeAdjust/VIPR/R2Rt/R2LtSt_BkReclnUpwdDnwd_Lt_Step1 ==
  note: // CurPosV 为0时表示有效，为1时表示无效，数据库中是这么定义的
  MSM_Trig : Inport
  Ena1 : Inport  Port=2
  Ena3 : Inport  Port=3
  Current_Pos : Inport  Port=4
  Calib_Min : Inport  Port=5
  Calib_Max : Inport  Port=6
  Tar_Pos : Inport  Port=7
  Tar_PosDelta : Inport  Port=8
  PosValid : Inport  Port=9
  ChildLocker : Inport  Port=10
  InvalidValue : Inport  Port=11
  Tick : Inport  Port=12
  CheckFinishTm : Inport  Port=13
  StConfig : Inport  Port=14
  InPosJdgModify : Lib/InPosJdgModify  SystemSampleTime=-1
  NOT : Logic  Operator=NOT  AllPortsSameDT=off  OutDataTypeStr=boolean
  OR : Logic  Operator=OR  AllPortsSameDT=off  OutDataTypeStr=boolean
  PA_KeSMSuMdRetryTm1_Val : Constant  Value=KeSMSuMdRetryTm1_Val
  PA_KeSMSwDltTrgtPos_Val1 : Constant  Value=0  OutDataTypeStr=boolean
  PA_KeSMSwDltTrgtPos_Val2 : Constant  Value=0  OutDataTypeStr=boolean
  Stg_judg : Lib/CommonUsed/Stg_judg  SystemSampleTime=-1
  Stg_judg1 : Lib/CommonUsed/Stg_judg  SystemSampleTime=-1
  Switch1 : Switch  Criteria=u2 > Threshold
  Switch4 : Switch  Criteria=u2 > Threshold
  isArrivedTarPos1 : Lib/CommonUsed/Subsystem  SystemSampleTime=-1
  ini_st : Outport
  ini_ReclnOverUp : Outport  Port=2
  ini_ReclnOverDwn : Outport  Port=3
  isArrivedTarPos : Outport  Port=4
  TarPos : Outport  Port=5
  Stg_done1 : Outport  Port=6
  Stg_done3 : Outport  Port=7
  wires:
  PA_KeSMSwDltTrgtPos_Val1/1 -> Stg_judg1/10
  CheckFinishTm/1 -> isArrivedTarPos1/4
  [InvalidValue] -> Switch1/3
  [TarPos3] -> Switch1/1
  [Ena3] -> Switch1/2
  Switch1/1 -> Switch4/3
  [TarPos1] -> Switch4/1
  [Ena1] -> Switch4/2
  Switch4/1 -> TarPos/1
  Stg_judg1/1 -> [TarPos3]
  Stg_judg/1 -> [TarPos1]
  Stg_judg1/2 -> Stg_done3/1, [Stgdone3]
  [Valid] -> Stg_judg1/8
  [isArrivedTarPos] -> Stg_judg1/7
  [ChildLocker] -> Stg_judg1/6
  [FrstJudgDone] -> Stg_judg1/5
  [tarPos] -> Stg_judg1/4
  [InvalidValue] -> Stg_judg1/3
  [Ena3] -> Stg_judg1/2
  Ena3/1 -> [Ena3]
  InPosJdgModify/2 -> ini_ReclnOverDwn/1
  InPosJdgModify/3 -> [ini_ReclnOverUp], ini_ReclnOverUp/1
  [isArrivedTarPos] -> Stg_judg/7
  [ChildLocker] -> Stg_judg/6
  [InvalidValue] -> Stg_judg/3
  [Ena1] -> Stg_judg/2
  Stg_judg/2 -> Stg_done1/1, [Stgdone1]
  Tick/1 -> Stg_judg/1, Stg_judg1/1
  isArrivedTarPos1/1 -> [isArrivedTarPos], isArrivedTarPos/1
  Tar_PosDelta/1 -> InPosJdgModify/5, isArrivedTarPos1/3
  Tar_Pos/1 -> Stg_judg/4, [tarPos], isArrivedTarPos1/2
  InPosJdgModify/1 -> ini_st/1, [FrstJudgDone]
  Calib_Max/1 -> InPosJdgModify/4
  Calib_Min/1 -> InPosJdgModify/3
  MSM_Trig/1 -> InPosJdgModify/1
  Current_Pos/1 -> InPosJdgModify/2, Stg_judg1/9, Stg_judg/9, isArrivedTarPos1/1
  PosValid/1 -> Stg_judg/8, [Valid]
  ChildLocker/1 -> [ChildLocker]
  Ena1/1 -> [Ena1]
  InvalidValue/1 -> [InvalidValue]
  StConfig/1 -> [StConfig], Stg_judg/11
  [StConfig] -> Stg_judg1/11
  [ini_ReclnOverUp] -> NOT/1
  PA_KeSMSwDltTrgtPos_Val2/1 -> Stg_judg/10
  OR/1 -> Stg_judg/5
  [FrstJudgDone] -> OR/2
  NOT/1 -> OR/1
  [CntLow] -> Stg_judg/12
  [CntLow] -> Stg_judg1/12
  PA_KeSMSuMdRetryTm1_Val/1 -> [CntLow]

== stateflow chart ModeAdjust/ModeAdjustRunnable_sys/ModeAdjust/LugL/Chart1 ==
  (default) -> (junction 1)
  (junction 1) -> (junction 3) [order 1] : [(Left_Done)]
  (junction 1) -> (junction 7) [order 2] : {
      | IfVeSMSbThdRwLtStRclCmdSrv_Val_write=IfVeSMSbThdRwLtStRclCmdSrv_Val_writeRaw;
      | Md_L_DoneOk=false;
      | Md_L_DoneFailed=false;
      | }
  (junction 3) -> (junction 5) : {
      | IfVeSMSbThdRwLtStRclCmdSrv_Val_write=false;
      | Md_L_DoneOk=Md_L_DoneOkRaw;
      | Md_L_DoneFailed=Md_L_DoneFailedRaw;
      | }
  (junction 5) -> (junction 7)
  (junction 7) -> (junction 46)
  data: Left_Done input boolean; IfVeSMSbThdRwLtStRclCmdSrv_Val_write output boolean; IfVeSMSbThdRwLtStRclCmdSrv_Val_writeRaw input; Md_L_DoneOkRaw input; Md_L_DoneFailedRaw input; Md_L_DoneOk output boolean; Md_L_DoneFailed output boolean

== stateflow chart ModeAdjust/ModeAdjustRunnable_sys/ModeAdjust/LugR/Chart ==
  (default) -> (junction 24)
  (junction 24) -> (junction 26) [order 1] : [!R3Rt_Step1_ini]
  (junction 26) -> (junction 71) [order 1] : [R3Rt_Step1_done]
  (junction 24) -> (junction 75) [order 2] : {R3Rt_Step1En=false;}
  (junction 26) -> (junction 28) [order 2] : {R3Rt_Step1En=true;}
  (junction 71) -> (junction 73) : {R3Rt_Step1En=false;}
  (junction 28) -> (junction 75)
  (junction 73) -> (junction 28)
  (junction 75) -> (junction 78)
  (junction 78) -> (junction 80) [order 1] : [(!R3Rt_Step2_ini)&&(R3Rt_Step1_done)]
  (junction 80) -> (junction 83) [order 1] : [R3Rt_Step2_done]
  (junction 78) -> (junction 30) [order 2] : {R3Rt_Step2En=false;}
  (junction 80) -> (junction 87) [order 2] : {R3Rt_Step2En=true;}
  (junction 83) -> (junction 85) : {R3Rt_Step2En=false;}
  (junction 87) -> (junction 30)
  (junction 85) -> (junction 87)
  data: R3Rt_Step1_ini input boolean; R3Rt_Step2_ini input boolean; R3Rt_Step1_done input boolean; R3Rt_Step2_done input boolean; R3Rt_Step1En output boolean; R3Rt_Step2En output boolean

== stateflow chart ModeAdjust/ModeAdjustRunnable_sys/ModeAdjust/ArrivedAtTargetPosChk/VIP/Drv/FtTargtCal ==
  (default) -> (junction 4)
  (junction 4) -> (junction 6) : {
      | FtTargetAngle = KeSMSuSecRwStVIPFtrstRefAngle-BkReclnUpwdDnwdPos/4000*78;
      | }
  (junction 6) -> (junction 9) [order 1] : [FtTargetAngle<0]
  (junction 6) -> (junction 13) [order 2]
  (junction 9) -> (junction 11) : {
      | FtTargetAngle=0;
      | }
  (junction 11) -> (junction 13)
  (junction 13) -> (junction 16)
  (junction 16) -> (junction 18) [order 1] : [FtTargetAngle>=108.2216]
  (junction 16) -> (junction 25) [order 2] : {
      | n=(sqrt(26933.84-(cos(FtTargetAngle*3.14159/180+0.43)*8110))-139.91)/0.12;
      | }
  (junction 18) -> (junction 20) : {
      | FtTargetPos=4000;
      | }
  (junction 25) -> (junction 28) : {
      | tmpTargetPos = n*4000;
      | tmpTargetPos = tmpTargetPos/335.245;
      | FtTargetPos = tmpTargetPos;
      | }
  (junction 20) -> (junction 28)
  (junction 28) -> (junction 32)
  data: BkReclnUpwdDnwdPos input single; KeSMSuSecRwStVIPFtrstRefAngle input single; FtTargetPos output uint16; FtTargetAngle local single; n local single; tmpTargetPos local single

== stateflow chart ModeAdjust/ModeAdjustRunnable_sys/ModeAdjust/LugR/Chart1 ==
  (default) -> (junction 10)
  (junction 10) -> (junction 36) [order 1] : [Right_Done]
  (junction 10) -> (junction 40) [order 2] : {
      | IfVeSMSbThdRwRtStRclCmdSrv_Val_write=IfVeSMSbThdRwRtStRclCmdSrv_Val_writeRaw;
      | Md_R_DoneOk=false;
      | Md_R_DoneFailed=false;
      | }
  (junction 36) -> (junction 38) : {
      | IfVeSMSbThdRwRtStRclCmdSrv_Val_write=false;
      | Md_R_DoneOk=Md_R_DoneOkRaw;
      | Md_R_DoneFailed=Md_R_DoneFailedRaw;
      | }
  (junction 38) -> (junction 40)
  (junction 40) -> (junction 43)
  data: Right_Done input boolean; IfVeSMSbThdRwRtStRclCmdSrv_Val_write output boolean; IfVeSMSbThdRwRtStRclCmdSrv_Val_writeRaw input; Md_R_DoneOkRaw input; Md_R_DoneFailedRaw input; Md_R_DoneOk output boolean; Md_R_DoneFailed output boolean

== stateflow chart ModeAdjust/ModeAdjustRunnable_sys/ModeAdjust/AcsMdEntry/Chart ==
  (default) -> (junction 10)
  (junction 10) -> (junction 58) [order 1] : [!Stg1ini]
  (junction 58) -> (junction 25) [order 1] : [Stg1done]
  (junction 10) -> (junction 26) [order 2] : {Stg1Req=false;}
  (junction 58) -> (junction 35) [order 2] : {Stg1Req=true;}
  (junction 25) -> (junction 18) : {
      | Stg1Req=false;
      | }
  (junction 35) -> (junction 26)
  (junction 18) -> (junction 35)
  (junction 26) -> (junction 36)
  (junction 36) -> (junction 44) [order 1] : [!Stg2ini]
  (junction 44) -> (junction 33) [order 1] : [Stg2done]
  (junction 36) -> (junction 27) [order 2] : {
      | Stg2Req=false;
      | }
  (junction 44) -> (junction 45) [order 2] : {
      | Stg2Req=true;
      | }
  (junction 33) -> (junction 73) : {
      | Stg2Req=false;
      | }
  (junction 45) -> (junction 27)
  (junction 73) -> (junction 45)
  (junction 27) -> (junction 42)
  (junction 42) -> (junction 28) [order 1] : [!Stg3ini]
  (junction 28) -> (junction 13) [order 1] : [Stg3done]
  (junction 42) -> (junction 56) [order 2] : {
      | Stg3Req=false;
      | }
  (junction 28) -> (junction 50) [order 2] : {
      | Stg3Req=true;
      | }
  (junction 13) -> (junction 23) : {
      | Stg3Req=false;
      | }
  (junction 50) -> (junction 56)
  (junction 23) -> (junction 50)
  (junction 56) -> (junction 52)
  (junction 52) -> (junction 31)
  (junction 31) -> (junction 34) [order 1] : [Stg1Req==true]
  (junction 31) -> (junction 38) [order 2]
  (junction 34) -> (junction 47) : {
      | R3ST_right_Step1=true;
      | R3ST_left_Step1=true;
      | R2ST_right_Step1=true;
      | R2ST_left_Step1=true;
      | DrvST_Step1=true;
      | PassST_Step1=true;
      | R3ST_right_Step2=false;
      | R3ST_left_Step2=false;
      | R2ST_right_Step2=false;
      | R2ST_left_Step2=false;
      | DrvST_Step2=false;
      | PassST_Step2=false;
      | R3ST_right_Step3=false;
      | R3ST_left_Step3=false;
      | R2ST_right_Step3=false;
      | R2ST_left_Step3=false;
      | DrvST_Step3=false;
      | PassST_Step3=false;
      | }
  (junction 38) -> (junction 24) [order 1] : [Stg2Req==true]
  (junction 38) -> (junction 43) [order 2]
  (junction 24) -> (junction 72) : {
      | R3ST_right_Step1=false;
      | R3ST_left_Step1=false;
      | R2ST_right_Step1=false;
      | R2ST_left_Step1=false;
      | DrvST_Step1=false;
      | PassST_Step1=false;
      | R3ST_right_Step2=true;
      | R3ST_left_Step2=true;
      | R2ST_right_Step2=true;
      | R2ST_left_Step2=true;
      | DrvST_Step2=true;
      | PassST_Step2=true;
      | R3ST_right_Step3=false;
      | R3ST_left_Step3=false;
      | R2ST_right_Step3=false;
      | R2ST_left_Step3=false;
      | DrvST_Step3=false;
      | PassST_Step3=false;
      | }
  (junction 43) -> (junction 46) [order 1] : [Stg3Req==true]
  (junction 43) -> (junction 71) [order 2] : {
      | R3ST_right_Step1=false;
      | R3ST_left_Step1=false;
      | R2ST_right_Step1=false;
      | R2ST_left_Step1=false;
      | DrvST_Step1=false;
      | PassST_Step1=false;
      | R3ST_right_Step2=false;
      | R3ST_left_Step2=false;
      | R2ST_right_Step2=false;
      | R2ST_left_Step2=false;
      | DrvST_Step2=false;
      | PassST_Step2=false;
      | R3ST_right_Step3=false;
      | R3ST_left_Step3=false;
      | R2ST_right_Step3=false;
      | R2ST_left_Step3=false;
      | DrvST_Step3=false;
      | PassST_Step3=false;
      | }
  (junction 46) -> (junction 61) : {
      | R3ST_right_Step1=false;
      | R3ST_left_Step1=false;
      | R2ST_right_Step1=false;
      | R2ST_left_Step1=false;
      | DrvST_Step1=false;
      | PassST_Step1=false;
      | R3ST_right_Step2=false;
      | R3ST_left_Step2=false;
      | R2ST_right_Step2=false;
      | R2ST_left_Step2=false;
      | DrvST_Step2=false;
      | PassST_Step2=false;
      | R3ST_right_Step3=true;
      | R3ST_left_Step3=true;
      | R2ST_right_Step3=false;
      | R2ST_left_Step3=false;
      | DrvST_Step3=false;
      | PassST_Step3=false;
      | }
  (junction 61) -> (junction 71)
  (junction 72) -> (junction 61)
  (junction 47) -> (junction 72)
  (junction 71) -> (junction 48)
  data: Stg1ini input boolean; Stg2ini input boolean; Stg3ini input boolean; Stg1done input boolean; Stg2done input boolean; Stg3done input boolean; Stg1Req output boolean; Stg2Req output boolean; Stg3Req output boolean; R3ST_right_Step1 output boolean; R3ST_left_Step1 output boolean; R2ST_right_Step1 output boolean; R2ST_left_Step1 output boolean; DrvST_Step1 output boolean; PassST_Step1 output boolean; R3ST_right_Step2 output boolean; R3ST_left_Step2 output boolean; R2ST_right_Step2 output boolean; R2ST_left_Step2 output boolean; DrvST_Step2 output boolean; PassST_Step2 output boolean; R3ST_right_Step3 output boolean; R3ST_left_Step3 output boolean; R2ST_right_Step3 output boolean; R2ST_left_Step3 output boolean; DrvST_Step3 output boolean; PassST_Step3 output boolean

== stateflow chart ModeAdjust/ModeAdjustRunnable_sys/ModeAdjust/VIPR/Chart1 ==
  (default) -> (junction 10)
  (junction 10) -> (junction 37) [order 1] : [RightDone]
  (junction 10) -> (junction 36) [order 2] : {
      | IfVeSMSbThdRwRtStRclCmdSrv_Val_write=IfVeSMSbThdRwRtStRclCmdSrv_Val_writeRaw;
      | IfVeSMSbThdRwLtStRclCmdSrv_Val_write=IfVeSMSbThdRwLtStRclCmdSrv_Val_writeRaw;
      | IfVeSMSbSecRwRtStRclCmdSrv_Val_write=IfVeSMSbSecRwRtStRclCmdSrv_Val_writeRaw;
      | IfVeSMSuPassStRclCmdSrv_Val_write=IfVeSMSuPassStRclCmdSrv_Val_writeRaw;
      | Md_R_DoneOk=false;
      | Md_R_DoneFailed=false;
      |
      | }
  (junction 37) -> (junction 39) : {
      | IfVeSMSbThdRwRtStRclCmdSrv_Val_write=false;
      | IfVeSMSbThdRwLtStRclCmdSrv_Val_write=false;
      | IfVeSMSbSecRwRtStRclCmdSrv_Val_write=false;
      | IfVeSMSuPassStRclCmdSrv_Val_write=false;
      | Md_R_DoneOk=Md_R_DoneOkRaw;
      | Md_R_DoneFailed=Md_R_DoneFailedRaw;
      | }
  (junction 39) -> (junction 36)
  (junction 36) -> (junction 43)
  data: RightDone input boolean; IfVeSMSbThdRwRtStRclCmdSrv_Val_write output boolean; IfVeSMSbSecRwRtStRclCmdSrv_Val_write output boolean; IfVeSMSbThdRwRtStRclCmdSrv_Val_writeRaw input; IfVeSMSbSecRwRtStRclCmdSrv_Val_writeRaw input; Md_R_DoneOkRaw input; Md_R_DoneFailedRaw input; Md_R_DoneOk output boolean; Md_R_DoneFailed output boolean; IfVeSMSbThdRwLtStRclCmdSrv_Val_writeRaw input; IfVeSMSbThdRwLtStRclCmdSrv_Val_write output boolean; IfVeSMSuPassStRclCmdSrv_Val_writeRaw input; IfVeSMSuPassStRclCmdSrv_Val_write output boolean

== stateflow chart ModeAdjust/ModeAdjustRunnable_sys/ModeAdjust/VIPR/Chart2 ==
  (default) -> (junction 450)
  (junction 450) -> (junction 448) [order 1] : [!L_R3Step1_ini]
  (junction 448) -> (junction 454) [order 1] : [L_R3Step1done]
  (junction 450) -> (junction 451) [order 2] : {L_R3Step1=false;}
  (junction 448) -> (junction 453) [order 2] : {L_R3Step1=true;}
  (junction 454) -> (junction 449) : {L_R3Step1=false;}
  (junction 453) -> (junction 451)
  (junction 449) -> (junction 453)
  (junction 451) -> (junction 552)
  (junction 552) -> (junction 563) [order 1] : [!R_R3Step1_ini]
  (junction 563) -> (junction 561) [order 1] : [R_R3Step1done]
  (junction 552) -> (junction 564) [order 2] : {R_R3Step1=false;}
  (junction 563) -> (junction 543) [order 2] : {R_R3Step1=true;}
  (junction 561) -> (junction 565) : {R_R3Step1=false;}
  (junction 543) -> (junction 564)
  (junction 565) -> (junction 543)
  (junction 564) -> (junction 441)
  (junction 441) -> (junction 444) [order 1] : [!L_R2Step1_ini&&L_PosOvrup]
  (junction 444) -> (junction 443) [order 1] : [L_R2Step1done]
  (junction 441) -> (junction 445) [order 2] : {L_R2Step1=false;}
  (junction 444) -> (junction 446) [order 2] : {L_R2Step1=true;}
  (junction 443) -> (junction 467) : {L_R2Step1=false;}
  (junction 446) -> (junction 445)
  (junction 467) -> (junction 446)
  (junction 445) -> (junction 460)
  (junction 460) -> (junction 455) [order 1] : [!L_R2Step2_ini&&L_R2Step1done]
  (junction 455) -> (junction 465) [order 1] : [L_R2Step2done]
  (junction 460) -> (junction 463) [order 2] : {L_R2Step2=false;}
  (junction 455) -> (junction 459) [order 2] : {L_R2Step2=true;}
  (junction 465) -> (junction 464) : {L_R2Step2=false;}
  (junction 459) -> (junction 463)
  (junction 464) -> (junction 459)
  (junction 463) -> (junction 577)
  (junction 577) -> (junction 581) [order 1] : [!L_R1Step1_ini&&Stage1_done]
  (junction 581) -> (junction 582) [order 1] : [Stage2_done]
  (junction 577) -> (junction 578) [order 2] : {L_R1Step1=false;}
  (junction 581) -> (junction 580) [order 2] : {L_R1Step1=true;}
  (junction 582) -> (junction 579) : {L_R1Step1=false;}
  (junction 580) -> (junction 578)
  (junction 579) -> (junction 580)
  (junction 578) -> (junction 466)
  (junction 466) -> (junction 456) [order 1] : [!L_R2Step3_ini&&Stage1_done&&Stage2_done]
  (junction 456) -> (junction 461) [order 1] : [Stage3_done]
  (junction 466) -> (junction 462) [order 2] : {L_R2Step3=false;}
  (junction 456) -> (junction 457) [order 2] : {L_R2Step3=true;}
  (junction 461) -> (junction 458) : {L_R2Step3=false;}
  (junction 457) -> (junction 462)
  (junction 458) -> (junction 457)
  (junction 462) -> (junction 473)
  data: R_R3Step1 output boolean; L_R3Step1 output boolean; L_R2Step1 output boolean; L_R2Step2 output boolean; L_R2Step3 output boolean; L_R3Step1_ini input boolean; L_R2Step1_ini input boolean; L_R2Step2_ini input boolean; L_R2Step3_ini input boolean; L_PosOvrup input boolean; L_R3Step1done input boolean; L_R2Step1done input boolean; L_R2Step2done input boolean; R_R3Step1_ini input boolean; R_R3Step1done input boolean; Stage1_done input boolean; Stage2_done input boolean; L_R1Step1_ini input boolean; L_R1Step1 output boolean; Stage3_done input boolean

== stateflow chart ModeAdjust/ModeAdjustRunnable_sys/ModeAdjust/RecoveryR/Chart ==
  (default) -> (junction 22)
  (junction 22) -> (junction 24) [order 1] : [!R2Rt_ini]
  (junction 24) -> (junction 26) [order 1] : [R2Rt_done]
  (junction 22) -> (junction 32) [order 2] : {R2Rt_En=false;}
  (junction 24) -> (junction 30) [order 2] : {R2Rt_En=true;}
  (junction 26) -> (junction 28) : {R2Rt_En=false;}
  (junction 30) -> (junction 32)
  (junction 28) -> (junction 30)
  (junction 32) -> (junction 69)
  (junction 69) -> (junction 73) [order 1] : [!PassSt_ini]
  (junction 73) -> (junction 67) [order 1] : [PassSt_done]
  (junction 69) -> (junction 74) [order 2] : {PassSt_En=false;}
  (junction 73) -> (junction 70) [order 2] : {PassSt_En=true;}
  (junction 67) -> (junction 71) : {PassSt_En=false;}
  (junction 70) -> (junction 74)
  (junction 71) -> (junction 70)
  data: R2Rt_ini input boolean; R2Rt_done input boolean; R2Rt_En output boolean; PassSt_ini input boolean; PassSt_done input boolean; PassSt_En output boolean

== stateflow chart ModeAdjust/ModeAdjustRunnable_sys/ModeAdjust/RecoveryR/Chart1 ==
  (default) -> (junction 10)
  (junction 10) -> (junction 36) [order 1] : [Right_Done]
  (junction 10) -> (junction 40) [order 2] : {
      | IfVeSMSbSecRwRtStRclCmdSrv_Val_write=IfVeSMSbSecRwRtStRclCmdSrv_Val_writeRaw;
      | IfVeSMSuPassStRclCmdSrv_Val_write=IfVeSMSuPassStRclCmdSrv_Val_writeRaw;
      | Md_R_DoneOk=false;
      | Md_R_DoneFailed=false;
      | }
  (junction 36) -> (junction 38) : {
      | IfVeSMSbSecRwRtStRclCmdSrv_Val_write=false;
      | IfVeSMSuPassStRclCmdSrv_Val_write=false;
      | Md_R_DoneOk=Md_R_DoneOkRaw;
      | Md_R_DoneFailed=Md_R_DoneFailedRaw;
      | }
  (junction 38) -> (junction 40)
  (junction 40) -> (junction 43)
  data: Right_Done input boolean; IfVeSMSbSecRwRtStRclCmdSrv_Val_write output boolean; IfVeSMSbSecRwRtStRclCmdSrv_Val_writeRaw input; Md_R_DoneOkRaw input; Md_R_DoneFailedRaw input; Md_R_DoneOk output boolean; Md_R_DoneFailed output boolean; IfVeSMSuPassStRclCmdSrv_Val_writeRaw input boolean; IfVeSMSuPassStRclCmdSrv_Val_write output boolean

== stateflow chart ModeAdjust/ModeAdjustRunnable_sys/ModeAdjust/OutNumR3_R ==
  (default) -> (junction 90) : {OutNum =0;}
  (junction 90) -> (junction 65) [order 1] : [HaltReq]
  (junction 90) -> (junction 66) [order 2]
  (junction 65) -> (junction 79)
  (junction 66) -> (junction 74) [order 1] : [EZE]
  (junction 66) -> (junction 83) [order 2]
  (junction 74) -> (junction 77) : {OutNum =1;}
  (junction 83) -> (junction 80) [order 1] : [(VIPR&&is6s7s)]
  (junction 83) -> (junction 81) [order 2]
  (junction 80) -> (junction 64) : {OutNum =2;}
  (junction 81) -> (junction 85) [order 1] : [Lug]
  (junction 81) -> (junction 89) [order 2]
  (junction 85) -> (junction 73) : {OutNum =3;}
  (junction 89) -> (junction 100) [order 1] : [FAMLY_L]
  (junction 89) -> (junction 51) [order 2]
  (junction 100) -> (junction 99) : {OutNum =4;}
  (junction 51) -> (junction 55) [order 1] : [FAMLY_R]
  (junction 51) -> (junction 52) [order 2]
  (junction 55) -> (junction 97) : {OutNum =5;}
  (junction 97) -> (junction 52)
  (junction 99) -> (junction 97)
  (junction 73) -> (junction 99)
  (junction 64) -> (junction 73)
  (junction 77) -> (junction 64)
  (junction 79) -> (junction 77)
  data: HaltReq input boolean; EZE input boolean; VIPR input boolean; Lug input boolean; FAMLY_L input boolean; OutNum output uint8; is6s7s input boolean; FAMLY_R input boolean
